simulink model "momentumBasedYoga"  (Simulink 8.8)
settings: Solver=FixedStepDiscrete  StartTime=0.0  StopTime="Config.SIMULATION_TIME "  FixedStep=Config.T_STEP  RelTol=1e-3  EnableMultiTasking=on
InitFcn:
  | cd(fileparts(which(bdroot)));
  | initMomentumBasedYoga;
StopFcn:
  | cd(fileparts(which(bdroot)));
  | stopMomentumBasedYoga;
undefined symbols (not defined in the file or in its folder): bVectorConstraints, Config, ConstraintsMatrix, Gain, Reg, ROBOT_DOF, ROBOT_DOF_FOR_SIMULINK, Sat, Sm
libraries: WBToolboxLibrary x89, simulink x4
(part 1 of 2)
settings Model: SuppressorTable=22 serialization::archive 11 0 6 0 0 0 11 0  Creator=daniele  LastModifiedBy=gnava
settings DataIOCC: SignalLoggingSaveFormat=Dataset
settings OptimizationCC: ExpressionDepthLimit=2147483647
settings DebuggingCC: SolverPrmCheckMsg=warning  AllowSymbolicDim=off
settings SFSimCC: SimParseCustomCode=off

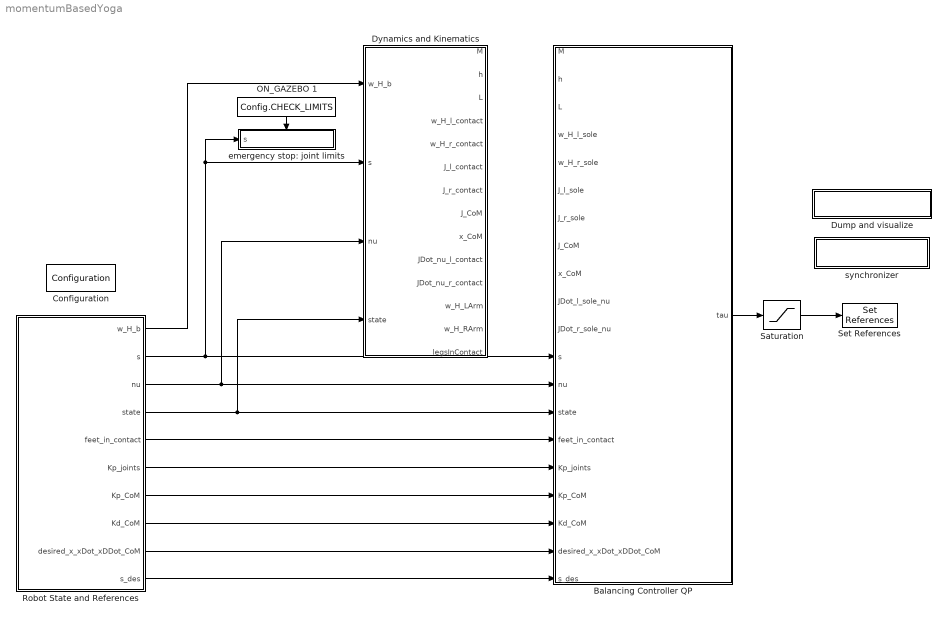
== system momentumBasedYoga ==
  Balancing Controller QP : Subsystem
  Configuration : WBToolboxLibrary/Utilities/Configuration  ConfigSource=Workspace  ConfigObject='WBTConfigRobot'  RobotName='icub'  UrdfFile='model.urdf'  ControlledJoints={'l_elbow','l_shoulder_pitch','torso_roll'}  ControlBoardsNames={'left_arm','right_arm','torso'}  LocalName='WBT'  GravityVector=[0,0,-9.81]
  Dump and visualize : Subsystem
      mask Display: disp('VISUALIZER')
  Dynamics and Kinematics : Subsystem
  ON_GAZEBO 1 : Constant  Value=Config.CHECK_LIMITS
  Robot State and References : Subsystem  Priority=-10
  Saturation : Saturate  UpperLimit=Sat.torque  LowerLimit=-Sat.torque
  Set References : WBToolboxLibrary/wholeBodyActuators/Set References  controlType=Torque  refSpeed=50
  emergency stop: joint limits : Subsystem
      mask Display: disp('EMERGENCY STOP')
  synchronizer : Subsystem
      mask Display: disp('SYNCHRONIZER')
  wires:
  Saturation/1 -> Set References/1
  ON_GAZEBO 1/1 -> emergency stop: joint limits/Enable
  Robot State and References/1(w_H_b) -> Dynamics and Kinematics/1(w_H_b)
  Robot State and References/2(s) -> Balancing Controller QP/12(s), emergency stop: joint limits/1(s), Dynamics and Kinematics/2(s)
  Robot State and References/3(nu) -> Balancing Controller QP/13(nu), Dynamics and Kinematics/3(nu)
  Robot State and References/4(state) -> Dynamics and Kinematics/4("state "), Balancing Controller QP/14(state)
  Robot State and References/5(feet_in_contact) -> Balancing Controller QP/15(feet_in_contact)
  Robot State and References/6(Kp_joints) -> Balancing Controller QP/16(Kp_joints)
  Robot State and References/7(Kp_CoM) -> Balancing Controller QP/17(Kp_CoM)
  Robot State and References/8(Kd_CoM) -> Balancing Controller QP/18(Kd_CoM)
  Robot State and References/9(desired_x_xDot_xDDot_CoM) -> Balancing Controller QP/19(desired_x_xDot_xDDot_CoM)
  Robot State and References/10(s_des) -> Balancing Controller QP/20(s_des)
  Balancing Controller QP/1("tau ") -> Saturation/1

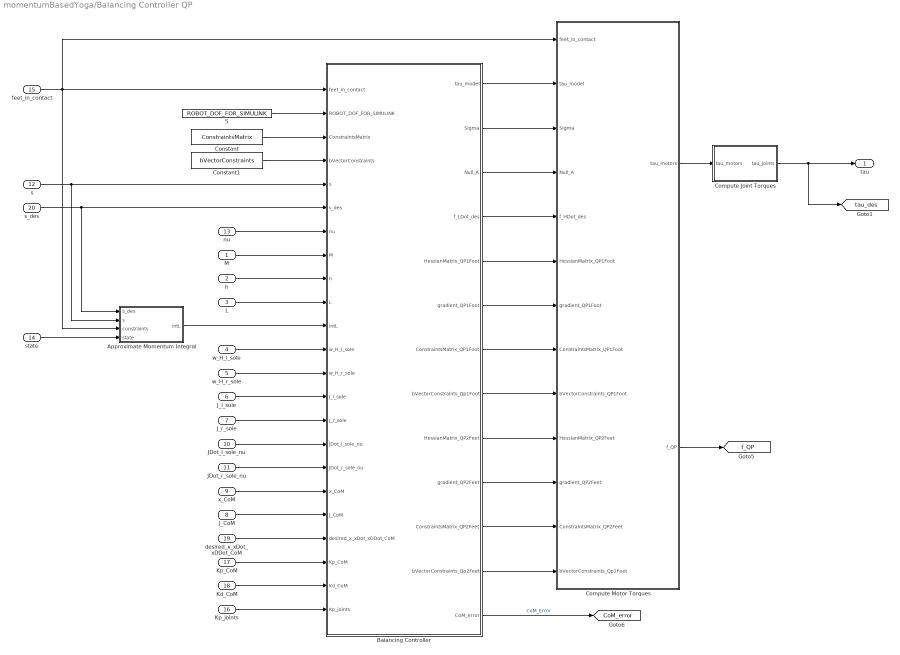
== system momentumBasedYoga/Balancing Controller QP ==
  M : Inport
  h : Inport  Port=2
  "L " : Inport  Port=3
  w_H_l_sole : Inport  Port=4
  w_H_r_sole : Inport  Port=5
  J_l_sole : Inport  Port=6
  J_r_sole : Inport  Port=7
  J_CoM : Inport  Port=8
  x_CoM : Inport  Port=9
  JDot_l_sole_nu : Inport  Port=10
  JDot_r_sole_nu : Inport  Port=11
  s : Inport  Port=12
  nu : Inport  Port=13
  state : Inport  Port=14
  feet_in_contact : Inport  Port=15
  Kp_joints : Inport  Port=16
  Kp_CoM : Inport  Port=17
  Kd_CoM : Inport  Port=18
  desired_x_xDot_xDDot_CoM : Inport  Port=19
  s_des : Inport  Port=20
  "    5" : Constant  Value=ROBOT_DOF_FOR_SIMULINK
  Approximate Momentum Integral : Subsystem
  "Balancing Controller " : MATLAB Function  TreatAsAtomicUnit=on
  Compute Joint Torques : Subsystem
  Compute Motor Torques : Subsystem
  Constant : Constant  Value=ConstraintsMatrix
  Constant1 : Constant  Value=bVectorConstraints
  "tau " : Outport
  tag scope: CoM_error=global, f_QP=global, tau_des=global
  wires:
  feet_in_contact/1 -> Compute Motor Torques/1(feet_in_contact), "Balancing Controller "/1(feet_in_contact), Approximate Momentum Integral/3(constraints)
  s/1 -> Approximate Momentum Integral/2(s), "Balancing Controller "/5(s)
  s_des/1 -> Approximate Momentum Integral/1(s_des), "Balancing Controller "/6(s_des)
  M/1 -> "Balancing Controller "/8(M)
  h/1 -> "Balancing Controller "/9(h)
  desired_x_xDot_xDDot_CoM/1 -> "Balancing Controller "/20(desired_x_xDot_xDDot_CoM)
  Kp_joints/1 -> "Balancing Controller "/23(Kp_joints)
  "L "/1 -> "Balancing Controller "/10(L)
  "    5"/1 -> "Balancing Controller "/2(ROBOT_DOF_FOR_SIMULINK)
  Constant/1 -> "Balancing Controller "/3(ConstraintsMatrix)
  Constant1/1 -> "Balancing Controller "/4(bVectorConstraints)
  nu/1 -> "Balancing Controller "/7(nu)
  Kp_CoM/1 -> "Balancing Controller "/21(Kp_CoM)
  Kd_CoM/1 -> "Balancing Controller "/22(Kd_CoM)
  w_H_r_sole/1 -> "Balancing Controller "/13(w_H_r_sole)
  w_H_l_sole/1 -> "Balancing Controller "/12(w_H_l_sole)
  J_l_sole/1 -> "Balancing Controller "/14(J_l_sole)
  J_r_sole/1 -> "Balancing Controller "/15(J_r_sole)
  Approximate Momentum Integral/1(intL) -> "Balancing Controller "/11(intL)
  JDot_l_sole_nu/1 -> "Balancing Controller "/16(JDot_l_sole_nu)
  JDot_r_sole_nu/1 -> "Balancing Controller "/17(JDot_r_sole_nu)
  J_CoM/1 -> "Balancing Controller "/19(J_CoM)
  x_CoM/1 -> "Balancing Controller "/18(x_CoM)
  state/1 -> Approximate Momentum Integral/4(state)
  Compute Motor Torques/1("tau_motors ") -> Compute Joint Torques/1(tau_motors)
  "Balancing Controller "/1(tau_model) -> Compute Motor Torques/2(tau_model)
  "Balancing Controller "/2(Sigma) -> Compute Motor Torques/3(Sigma)
  "Balancing Controller "/3(Null_A) -> Compute Motor Torques/4(Null_A)
  "Balancing Controller "/4(f_LDot_des) -> Compute Motor Torques/5(f_HDot_des)
  "Balancing Controller "/5(HessianMatrix_QP1Foot) -> Compute Motor Torques/6(HessianMatrix_QP1Foot)
  "Balancing Controller "/6(gradient_QP1Foot) -> Compute Motor Torques/7(gradient_QP1Foot)
  "Balancing Controller "/7(ConstraintsMatrix_QP1Foot) -> Compute Motor Torques/8(ConstraintsMatrix_QP1Foot)
  "Balancing Controller "/8(bVectorConstraints_Qp1Foot) -> Compute Motor Torques/9(bVectorConstraints_QP1Foot)
  "Balancing Controller "/9(HessianMatrix_QP2Feet) -> Compute Motor Torques/10(HessianMatrix_QP2Feet)
  "Balancing Controller "/10(gradient_QP2Feet) -> Compute Motor Torques/11(gradient_QP2Feet)
  "Balancing Controller "/11(ConstraintsMatrix_QP2Feet) -> Compute Motor Torques/12(ConstraintsMatrix_QP2Feet)
  "Balancing Controller "/12(bVectorConstraints_Qp2Feet) -> Compute Motor Torques/13(bVectorConstraints_Qp2Feet)
  "Balancing Controller "/13(CoM_error) -> [CoM_error]  "CoM_Error"
  Compute Motor Torques/2(f_QP) -> [f_QP]
  Compute Joint Torques/1(tau_joints) -> "tau "/1, [tau_des]

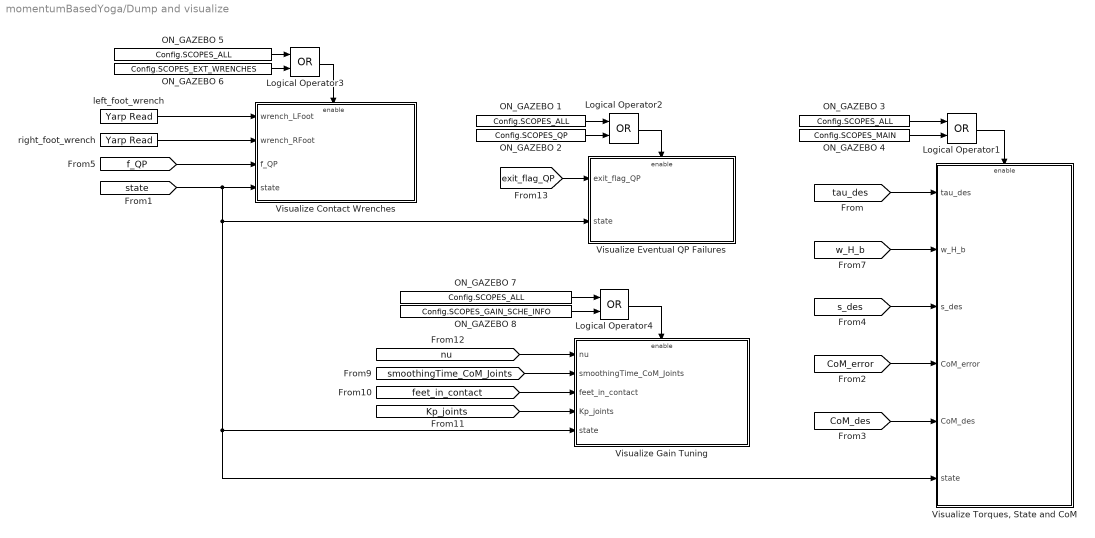
== system momentumBasedYoga/Dump and visualize ==
  Logical Operator{1..4} (4 alike) : Logic  Operator=OR  AllPortsSameDT=off  OutDataTypeStr=boolean
  ON_GAZEBO {1,3,5,7} (4 alike) : Constant  Value=Config.SCOPES_ALL
  ON_GAZEBO 2 : Constant  Value=Config.SCOPES_QP
  ON_GAZEBO 4 : Constant  Value=Config.SCOPES_MAIN
  ON_GAZEBO 6 : Constant  Value=Config.SCOPES_EXT_WRENCHES
  ON_GAZEBO 8 : Constant  Value=Config.SCOPES_GAIN_SCHE_INFO
  Visualize Contact Wrenches : Subsystem
  Visualize Eventual QP Failures : Subsystem
  "Visualize Gain Tuning  " : Subsystem
  "Visualize Torques, State and CoM" : Subsystem
  left_foot_wrench : WBToolboxLibrary/Utilities/Yarp Read  portName=Ports.WRENCH_LEFT_FOOT  signalSize=6  timeout=0.5  blocking=off  timestamp=off  autoconnect=on  errorOnConnection=on
  right_foot_wrench : WBToolboxLibrary/Utilities/Yarp Read  portName=Ports.WRENCH_RIGHT_FOOT  signalSize=6  timeout=0.5  blocking=off  timestamp=off  autoconnect=on  errorOnConnection=on
  wires:
  ON_GAZEBO 3/1 -> Logical Operator1/1
  ON_GAZEBO 4/1 -> Logical Operator1/2
  Logical Operator1/1 -> "Visualize Torques, State and CoM"/Enable
  [CoM_error] -> "Visualize Torques, State and CoM"/4(CoM_error)
  [s_des] -> "Visualize Torques, State and CoM"/3(s_des)
  [w_H_b] -> "Visualize Torques, State and CoM"/2(w_H_b)
  [tau_des] -> "Visualize Torques, State and CoM"/1(tau_des)
  [CoM_des] -> "Visualize Torques, State and CoM"/5(CoM_des)
  right_foot_wrench/1 -> Visualize Contact Wrenches/2(wrench_RFoot)
  [exit_flag_QP] -> Visualize Eventual QP Failures/1(exit_flag_QP)
  Logical Operator2/1 -> Visualize Eventual QP Failures/Enable
  ON_GAZEBO 1/1 -> Logical Operator2/1
  ON_GAZEBO 2/1 -> Logical Operator2/2
  ON_GAZEBO 5/1 -> Logical Operator3/1
  ON_GAZEBO 6/1 -> Logical Operator3/2
  [f_QP] -> Visualize Contact Wrenches/3(f_QP)
  ON_GAZEBO 7/1 -> Logical Operator4/1
  Logical Operator4/1 -> "Visualize Gain Tuning  "/Enable
  ON_GAZEBO 8/1 -> Logical Operator4/2
  [nu] -> "Visualize Gain Tuning  "/1(nu)
  [Kp_joints] -> "Visualize Gain Tuning  "/4(Kp_joints)
  [feet_in_contact] -> "Visualize Gain Tuning  "/3(feet_in_contact)
  [smoothingTime_CoM_Joints] -> "Visualize Gain Tuning  "/2(smoothingTime_CoM_Joints)
  [state] -> "Visualize Torques, State and CoM"/6(state), "Visualize Gain Tuning  "/5(state), Visualize Eventual QP Failures/2(state), Visualize Contact Wrenches/4(state)
  Logical Operator3/1 -> Visualize Contact Wrenches/Enable
  left_foot_wrench/1 -> Visualize Contact Wrenches/1(wrench_LFoot)

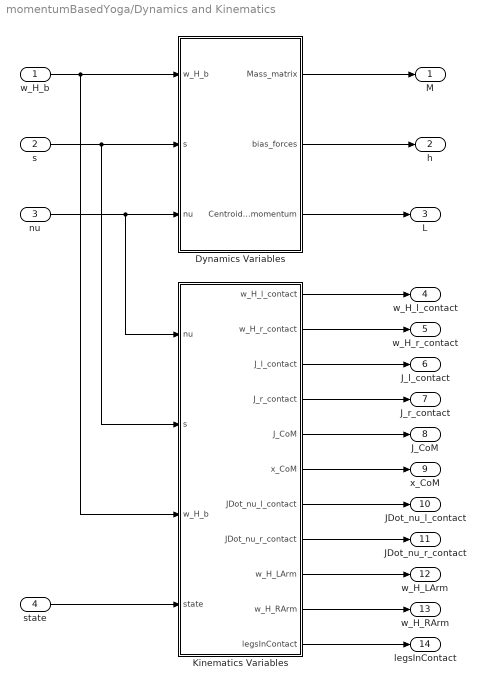
== system momentumBasedYoga/Dynamics and Kinematics ==
  w_H_b : Inport
  s : Inport  Port=2
  nu : Inport  Port=3
  "state " : Inport  Port=4
  Dynamics Variables : Subsystem
  Kinematics Variables : Subsystem
  M : Outport
  h : Outport  Port=2
  L : Outport  Port=3
  w_H_l_contact : Outport  Port=4
  w_H_r_contact : Outport  Port=5
  J_l_contact : Outport  Port=6
  J_r_contact : Outport  Port=7
  J_CoM : Outport  Port=8
  x_CoM : Outport  Port=9
  JDot_nu_l_contact : Outport  Port=10
  JDot_nu_r_contact : Outport  Port=11
  w_H_LArm : Outport  Port=12
  w_H_RArm : Outport  Port=13
  legsInContact : Outport  Port=14
  wires:
  Dynamics Variables/1(Mass_matrix) -> M/1
  Dynamics Variables/2(bias_forces) -> h/1
  Dynamics Variables/3(Centroidal_momentum) -> L/1
  Kinematics Variables/4(J_r_contact) -> J_r_contact/1
  Kinematics Variables/3(J_l_contact) -> J_l_contact/1
  "state "/1 -> Kinematics Variables/4("state ")
  Kinematics Variables/7(JDot_nu_l_contact) -> JDot_nu_l_contact/1
  Kinematics Variables/8(JDot_nu_r_contact) -> JDot_nu_r_contact/1
  Kinematics Variables/10(w_H_RArm) -> w_H_RArm/1
  Kinematics Variables/5(J_CoM) -> J_CoM/1
  Kinematics Variables/1(w_H_l_contact) -> w_H_l_contact/1
  w_H_b/1 -> Kinematics Variables/3(w_H_b), Dynamics Variables/1(w_H_b)
  Kinematics Variables/6(x_CoM) -> x_CoM/1
  Kinematics Variables/2(w_H_r_contact) -> w_H_r_contact/1
  nu/1 -> Kinematics Variables/1(nu), Dynamics Variables/3(nu)
  Kinematics Variables/11(legsInContact) -> legsInContact/1
  Kinematics Variables/9(w_H_LArm) -> w_H_LArm/1
  s/1 -> Kinematics Variables/2(s), Dynamics Variables/2(s)

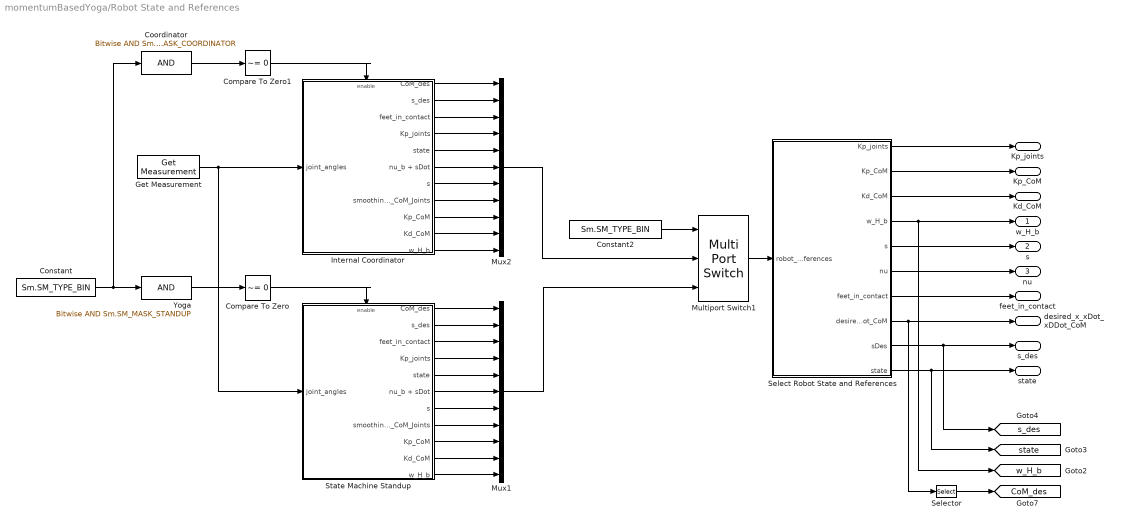
== system momentumBasedYoga/Robot State and References ==
  Compare To Zero : simulink/Logic and Bit Operations/Compare To Zero  relop=~=  OutDataTypeStr=boolean
  Compare To Zero1 : simulink/Logic and Bit Operations/Compare To Zero  relop=~=  OutDataTypeStr=boolean
  Constant : Constant  Priority=-10  Value=Sm.SM_TYPE_BIN  OutDataTypeStr=uint8
  Constant2 : Constant  Priority=-10  Value=Sm.SM_TYPE_BIN  OutDataTypeStr=uint8
  Coordinator : simulink/Logic and Bit Operations/Bitwise Operator  logicop=AND  UseBitMask=on  BitMask=Sm.SM_MASK_COORDINATOR  BitMaskRealWorld=Stored Integer
  Get Measurement : WBToolboxLibrary/wholeBodyStates/Get Measurement  measuredType=Joints Position
  Internal Coordinator : Subsystem
  Multiport Switch1 : MultiPortSwitch  DataPortOrder=Specify indices  DataPortIndices={1, 2}
  Mux1 : Mux  Inputs=11
  Mux2 : Mux  Inputs=11
  Select Robot State and References : Subsystem
  Selector : Selector  NumberOfDimensions=2  InputPortWidth=3  IndexOptions=Index vector (dialog),Index vector (dialog)  Indices=[1 2 3],[1]  OutputSizes=1,1
  State Machine Standup : Subsystem  Priority=-100
  Yoga : simulink/Logic and Bit Operations/Bitwise Operator  logicop=AND  UseBitMask=on  BitMask=Sm.SM_MASK_STANDUP  BitMaskRealWorld=Stored Integer
  w_H_b : Outport
  s : Outport  Port=2
  nu : Outport  Port=3
  state : Outport  Port=4
  feet_in_contact : Outport  Port=5
  Kp_joints : Outport  Port=6
  Kp_CoM : Outport  Port=7
  Kd_CoM : Outport  Port=8
  desired_x_xDot_xDDot_CoM : Outport  Port=9
  s_des : Outport  Port=10
  tag scope: CoM_des=global, s_des=global, state=global, w_H_b=global
  wires:
  Constant/1 -> Yoga/1, Coordinator/1
  State Machine Standup/3(feet_in_contact) -> Mux1/3
  State Machine Standup/2(s_des) -> Mux1/2
  State Machine Standup/1(CoM_des) -> Mux1/1
  Internal Coordinator/1(CoM_des) -> Mux2/1
  Internal Coordinator/2(s_des) -> Mux2/2
  Internal Coordinator/3(feet_in_contact) -> Mux2/3
  State Machine Standup/4(Kp_joints) -> Mux1/4
  Internal Coordinator/4(Kp_joints) -> Mux2/4
  State Machine Standup/5(state) -> Mux1/5
  Internal Coordinator/5(state) -> Mux2/5
  Internal Coordinator/6(nu_b + sDot) -> Mux2/6
  Internal Coordinator/7(s) -> Mux2/7
  State Machine Standup/6(nu_b + sDot) -> Mux1/6
  State Machine Standup/7(s) -> Mux1/7
  Coordinator/1 -> Compare To Zero1/1
  Yoga/1 -> Compare To Zero/1
  Compare To Zero/1 -> State Machine Standup/Enable
  Compare To Zero1/1 -> Internal Coordinator/Enable
  Internal Coordinator/8(smoothingTime_CoM_Joints) -> Mux2/8
  State Machine Standup/8(smoothingTime_CoM_Joints) -> Mux1/8
  State Machine Standup/9(Kp_CoM) -> Mux1/9
  State Machine Standup/10(Kd_CoM) -> Mux1/10
  Internal Coordinator/9(Kp_CoM) -> Mux2/9
  Internal Coordinator/10(Kd_CoM) -> Mux2/10
  Constant2/1 -> Multiport Switch1/1
  Get Measurement/1 -> Internal Coordinator/1(joint_angles), State Machine Standup/1(joint_angles)
  State Machine Standup/11(w_H_b) -> Mux1/11
  Internal Coordinator/11(w_H_b) -> Mux2/11
  Mux2/1 -> Multiport Switch1/2
  Mux1/1 -> Multiport Switch1/3
  Multiport Switch1/1 -> Select Robot State and References/1(robot_state_and_references)
  Select Robot State and References/1(Kp_joints) -> Kp_joints/1
  Select Robot State and References/2(Kp_CoM) -> Kp_CoM/1
  Select Robot State and References/3(Kd_CoM) -> Kd_CoM/1
  Select Robot State and References/4(w_H_b) -> w_H_b/1, [w_H_b]
  Select Robot State and References/5(s) -> s/1
  Select Robot State and References/6(nu) -> nu/1
  Select Robot State and References/7(feet_in_contact) -> feet_in_contact/1
  Select Robot State and References/8(desired_x_xDot_xDDot_CoM) -> desired_x_xDot_xDDot_CoM/1, Selector/1
  Select Robot State and References/9(sDes) -> s_des/1, [s_des]
  Select Robot State and References/10(state) -> state/1, [state]
  Selector/1 -> [CoM_des]

== system momentumBasedYoga/emergency stop: joint limits ==
  s : Inport
  Enable : EnablePort
  Assertion : Assertion
  Get Limits : WBToolboxLibrary/wholeBodyStates/Get Limits  limitsSource=ControlBoard  limitsType=Position
  MATLAB Function : MATLAB Function  TreatAsAtomicUnit=on
  index1 : Constant  Value=0.01  VectorParams1D=off
  wires:
  Get Limits/1 -> MATLAB Function/1(umin)
  Get Limits/2 -> MATLAB Function/2(umax)
  index1/1 -> MATLAB Function/4(tol)
  s/1 -> MATLAB Function/3(u)
  MATLAB Function/1(inRange) -> Assertion/1

== system momentumBasedYoga/synchronizer ==
  GAZEBO_SYNCHRONIZER : Subsystem
  Logical Operator : Logic  Operator=NOT  AllPortsSameDT=off  OutDataTypeStr=boolean
  "ON_GAZEBO " : Constant  Value=Config.ON_GAZEBO
  REAL_TIME_SYNC : Subsystem
  wires:
  Logical Operator/1 -> REAL_TIME_SYNC/Enable
  "ON_GAZEBO "/1 -> GAZEBO_SYNCHRONIZER/Enable, Logical Operator/1

== system momentumBasedYoga/Balancing Controller QP/Approximate Momentum Integral ==
  s_des : Inport
  s : Inport  Port=2
  constraints : Inport  Port=3
  state : Inport  Port=4
  Centroidal Momentum : WBToolboxLibrary/wholeBodyModel/Dynamics/Centroidal Momentum
  Compute base to fixed link transform : Subsystem
  Jacobian : WBToolboxLibrary/wholeBodyModel/Jacobians/Jacobian  frameName=Frames.LEFT_FOOT
  Jacobian1 : WBToolboxLibrary/wholeBodyModel/Jacobians/Jacobian  frameName=Frames.RIGHT_FOOT
  References for L : MATLAB Function  TreatAsAtomicUnit=on
  Sum : Sum  Inputs=|-+
  Switch : Switch  Criteria=u2 > Threshold  Threshold=0.1
  choose base to world transform : MATLAB Function  TreatAsAtomicUnit=on
  inertial : WBToolboxLibrary/Utilities/Yarp Read  portName=Ports.IMU  signalSize=12  timeout=0.5  blocking=off  timestamp=off  autoconnect=on  errorOnConnection=on
  intL : Outport
  wires:
  s_des/1 -> Compute base to fixed link transform/1(s), Centroidal Momentum/2, Jacobian/2, Sum/1, Jacobian1/2
  s/1 -> Sum/2
  Sum/1 -> Centroidal Momentum/4, References for L/1(s_err)
  References for L/1(nu_b_equivalent) -> Centroidal Momentum/3
  Jacobian/1 -> References for L/2(JL)
  Centroidal Momentum/1 -> intL/1
  Jacobian1/1 -> References for L/3(JR)
  constraints/1 -> References for L/4(activeFeetConstraints)
  state/1 -> choose base to world transform/1(state)
  choose base to world transform/1(booleanState) -> Switch/2
  Switch/1 -> Centroidal Momentum/1, Jacobian/1, Jacobian1/1
  inertial/1 -> Compute base to fixed link transform/2(inertial)
  Compute base to fixed link transform/1(fixed_LFoot_H_b) -> Switch/1
  Compute base to fixed link transform/2(fixed_RFoot_H_b) -> Switch/3

== system momentumBasedYoga/Balancing Controller QP/Compute Joint Torques ==
  tau_motors : Inport
  " " : Constant  Value=Config.USE_MOTOR_REFLECTED_INERTIA
  "(transpose(T*Gamma))^{-1}*I_m*(T*Gamma)^{-1}" : MATLAB Function  TreatAsAtomicUnit=on
  Add : Sum  Inputs=-+
  Feedforward : Gain  Gain=Config.K_ff
  Get Measurement : WBToolboxLibrary/wholeBodyStates/Get Measurement  measuredType=Joints Acceleration
  Product : Product  Multiplication=Matrix(*)
  Switch : Switch  Criteria=u2 > Threshold
  tau_joints : Outport
  wires:
  Get Measurement/1 -> Product/2
  Product/1 -> Feedforward/1
  Feedforward/1 -> Add/1
  Add/1 -> Switch/1
  " "/1 -> Switch/2
  Switch/1 -> tau_joints/1
  tau_motors/1 -> Add/2, Switch/3
  "(transpose(T*Gamma))^{-1}*I_m*(T*Gamma)^{-1}"/1(reflectedInertia) -> Product/1

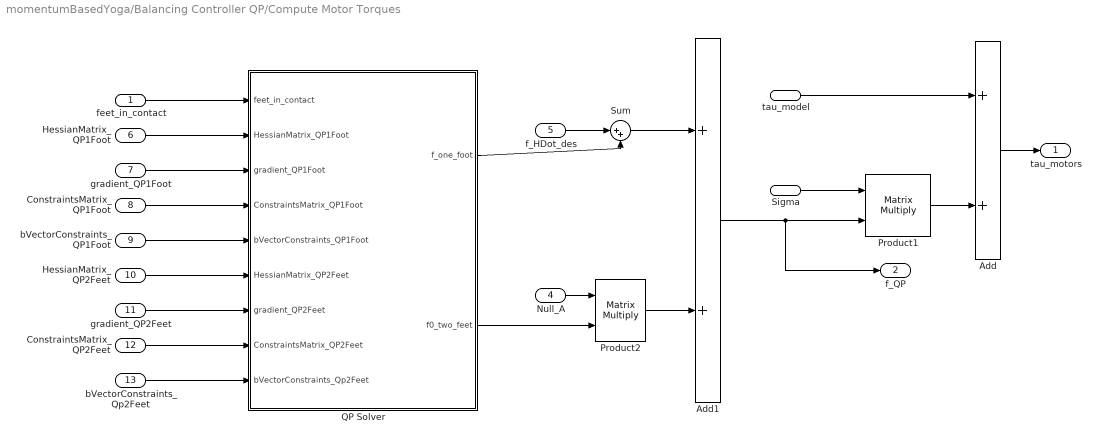
== system momentumBasedYoga/Balancing Controller QP/Compute Motor Torques ==
  feet_in_contact : Inport
  tau_model : Inport  Port=2
  Sigma : Inport  Port=3
  Null_A : Inport  Port=4
  f_HDot_des : Inport  Port=5
  HessianMatrix_QP1Foot : Inport  Port=6
  gradient_QP1Foot : Inport  Port=7
  ConstraintsMatrix_QP1Foot : Inport  Port=8
  bVectorConstraints_QP1Foot : Inport  Port=9
  HessianMatrix_QP2Feet : Inport  Port=10
  gradient_QP2Feet : Inport  Port=11
  ConstraintsMatrix_QP2Feet : Inport  Port=12
  bVectorConstraints_Qp2Feet : Inport  Port=13
  Add : Sum
  Add1 : Sum
  Product1 : Product  Multiplication=Matrix(*)
  Product2 : Product  Multiplication=Matrix(*)
  QP Solver : Subsystem
  Sum : Sum  Inputs=|++
  "tau_motors " : Outport
  f_QP : Outport  Port=2
  wires:
  Null_A/1 -> Product2/1
  QP Solver/1(f_one_foot) -> Sum/2
  Product1/1 -> Add/2
  tau_model/1 -> Add/1
  Add/1 -> "tau_motors "/1
  Add1/1 -> f_QP/1, Product1/2
  Sum/1 -> Add1/1
  Product2/1 -> Add1/2
  Sigma/1 -> Product1/1
  QP Solver/2(f0_two_feet) -> Product2/2
  gradient_QP1Foot/1 -> QP Solver/3(gradient_QP1Foot)
  ConstraintsMatrix_QP2Feet/1 -> QP Solver/8(ConstraintsMatrix_QP2Feet)
  feet_in_contact/1 -> QP Solver/1(feet_in_contact)
  bVectorConstraints_QP1Foot/1 -> QP Solver/5(bVectorConstraints_QP1Foot)
  HessianMatrix_QP1Foot/1 -> QP Solver/2(HessianMatrix_QP1Foot)
  ConstraintsMatrix_QP1Foot/1 -> QP Solver/4(ConstraintsMatrix_QP1Foot)
  gradient_QP2Feet/1 -> QP Solver/7(gradient_QP2Feet)
  HessianMatrix_QP2Feet/1 -> QP Solver/6(HessianMatrix_QP2Feet)
  bVectorConstraints_Qp2Feet/1 -> QP Solver/9(bVectorConstraints_Qp2Feet)
  f_HDot_des/1 -> Sum/1

== system momentumBasedYoga/Dump and visualize/Visualize Contact Wrenches ==
  wrench_LFoot : Inport
  wrench_RFoot : Inport  Port=2
  f_QP : Inport  Port=3
  state : Inport  Port=4
  Enable : EnablePort
  Demux{1..5} (5 alike) : Demux  Outputs=2
  Left Foot Forces : Scope  NumInputPorts=4
  Left Foot Moments : Scope  NumInputPorts=4
  Right Foot Forces : Scope  NumInputPorts=4
  Right Foot Moments : Scope  NumInputPorts=4
  Sum{1..4} (4 alike) : Sum  Inputs=+-|
  wires:
  f_QP/1 -> Demux1/1
  Demux1/1 -> Demux2/1  "LFoot_wrench"
  wrench_LFoot/1 -> Demux3/1  "LFoot_wrench"
  Sum2/1 -> Left Foot Moments/3  "moments error"
  Sum1/1 -> Left Foot Forces/3  "forces error"
  Demux2/1 -> Sum1/1, Left Foot Forces/1  "desired forces"
  Demux2/2 -> Sum2/1, Left Foot Moments/1  "desired moments"
  Demux3/1 -> Sum1/2, Left Foot Forces/2  "measured forces"
  Demux3/2 -> Left Foot Moments/2, Sum2/2  "measured moments"
  Demux4/2 -> Sum4/1, Right Foot Moments/1  "desired moments"
  Demux5/1 -> Sum3/2, Right Foot Forces/2  "measured forces"
  Demux4/1 -> Sum3/1, Right Foot Forces/1  "desired forces"
  Demux5/2 -> Right Foot Moments/2, Sum4/2  "measured moments"
  Sum3/1 -> Right Foot Forces/3  "forces error"
  Sum4/1 -> Right Foot Moments/3  "moments error"
  Demux1/2 -> Demux4/1  "RFoot_wrench"
  state/1 -> Left Foot Forces/4, Left Foot Moments/4, Right Foot Forces/4, Right Foot Moments/4
  wrench_RFoot/1 -> Demux5/1  "RFoot_wrench"

== system momentumBasedYoga/Dump and visualize/Visualize Eventual QP Failures ==
  exit_flag_QP : Inport
  state : Inport  Port=2
  Enable : EnablePort
  "QP status (0: no failure, 1: not using)" : Scope  NumInputPorts=2
  wires:
  exit_flag_QP/1 -> "QP status (0: no failure, 1: not using)"/1
  state/1 -> "QP status (0: no failure, 1: not using)"/2

== system momentumBasedYoga/Dump and visualize/Visualize Gain Tuning   ==
  nu : Inport
  smoothingTime_CoM_Joints : Inport  Port=2
  feet_in_contact : Inport  Port=3
  Kp_joints : Inport  Port=4
  state : Inport  Port=5
  Enable : EnablePort
  Demux : Demux  Outputs=2
  DoFs converter : WBToolboxLibrary/Utilities/DoFs converter  yarp2WBIOption=From YARP to WBI
  DoFs converter1 : WBToolboxLibrary/Utilities/DoFs converter  yarp2WBIOption=From YARP to WBI
  Feet in Contact : Scope
  Gain : Gain  Gain=180/pi
  Gain1 : Gain  Gain=180/pi
  Kp Joints : Scope  NumInputPorts=6
  Selector1 : Selector  InputPortWidth=6+ROBOT_DOF  IndexOptions=Index vector (dialog)  Indices=[7:6+ROBOT_DOF]  OutputSizes=1
  Selector2 : Selector  InputPortWidth=6+ROBOT_DOF  IndexOptions=Index vector (dialog)  Indices=[1:6]  OutputSizes=1
  nu_base : Scope  NumInputPorts=3
  sDot : Scope  NumInputPorts=6
  smoothingTime CoM and Joints : Scope  NumInputPorts=2
  wires:
  state/1 -> sDot/6, nu_base/3, Kp Joints/6, smoothingTime CoM and Joints/2
  feet_in_contact/1 -> Feet in Contact/1
  Kp_joints/1 -> DoFs converter/1
  smoothingTime_CoM_Joints/1 -> smoothingTime CoM and Joints/1
  DoFs converter/4 -> Kp Joints/4  "left_leg"
  DoFs converter/5 -> Kp Joints/5  "right_leg"
  DoFs converter/3 -> Kp Joints/3  "right_arm"
  DoFs converter/1 -> Kp Joints/1  "torso"
  DoFs converter/2 -> Kp Joints/2  "left_arm"
  Selector1/1 -> Gain/1
  DoFs converter1/4 -> sDot/4  "left_leg"
  DoFs converter1/3 -> sDot/3  "right_arm"
  DoFs converter1/1 -> sDot/1  "torso"
  DoFs converter1/2 -> sDot/2  "left_arm"
  nu/1 -> Selector2/1, Selector1/1
  Selector2/1 -> Demux/1
  Demux/1 -> nu_base/1  "v_b"
  Demux/2 -> Gain1/1
  Gain/1 -> DoFs converter1/1
  Gain1/1 -> nu_base/2  "omega_b"
  DoFs converter1/5 -> sDot/5  "right_leg"

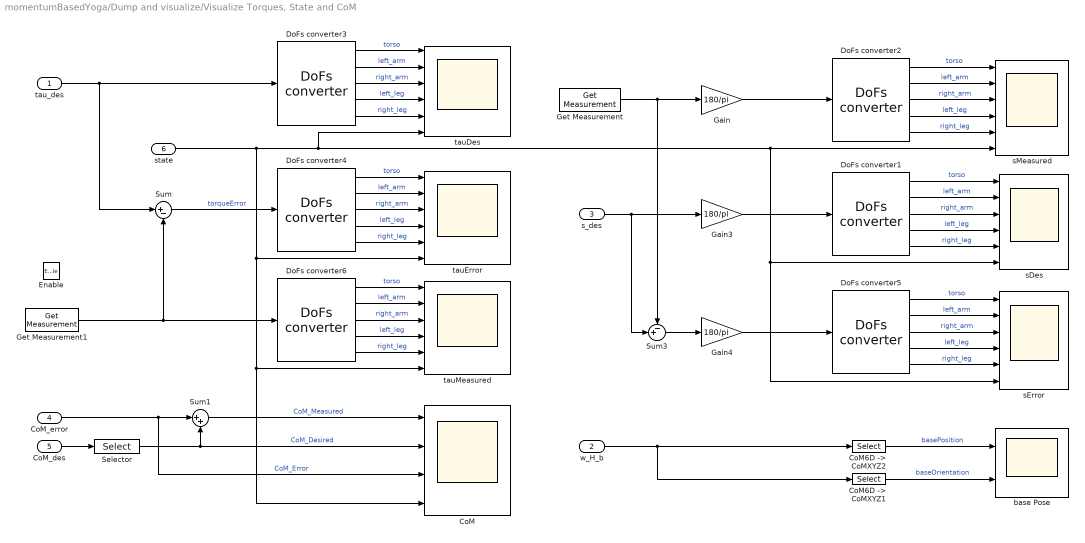
== system momentumBasedYoga/Dump and visualize/Visualize Torques, State and CoM ==
  tau_des : Inport
  w_H_b : Inport  Port=2
  s_des : Inport  Port=3
  CoM_error : Inport  Port=4
  CoM_des : Inport  Port=5
  state : Inport  Port=6
  Enable : EnablePort
  CoM : Scope  NumInputPorts=4
  "CoM6D ->  CoMXYZ1" : Selector  NumberOfDimensions=2  InputPortWidth=7  IndexOptions=Index vector (dialog),Index vector (dialog)  Indices=[1 2 3],[1 2 3]  OutputSizes=1,1
  "CoM6D ->  CoMXYZ2" : Selector  NumberOfDimensions=2  InputPortWidth=7  IndexOptions=Index vector (dialog),Index vector (dialog)  Indices=[1 2 3],[4]  OutputSizes=1,1
  DoFs converter{1..6} (6 alike) : WBToolboxLibrary/Utilities/DoFs converter  yarp2WBIOption=From YARP to WBI
  Gain : Gain  Gain=180/pi
  Gain3 : Gain  Gain=180/pi
  Gain4 : Gain  Gain=180/pi
  Get Measurement : WBToolboxLibrary/wholeBodyStates/Get Measurement  measuredType=Joints Position
  Get Measurement1 : WBToolboxLibrary/wholeBodyStates/Get Measurement  measuredType=Joints Torque
  Selector : Selector  NumberOfDimensions=2  IndexOptions=Index vector (dialog),Index vector (dialog)  Indices=[1:3],1  OutputSizes=1,1
  Sum : Sum  Inputs=|+-
  Sum1 : Sum  Inputs=|++
  Sum3 : Sum  Inputs=-+|
  base Pose : Scope  NumInputPorts=2
  sDes : Scope  NumInputPorts=6
  sError : Scope  NumInputPorts=6
  sMeasured : Scope  NumInputPorts=6
  tauDes : Scope  NumInputPorts=6
  tauError : Scope  NumInputPorts=6
  tauMeasured : Scope  NumInputPorts=6
  wires:
  CoM_error/1 -> Sum1/1, CoM/3  "CoM_Error"
  CoM_des/1 -> Selector/1
  Gain/1 -> DoFs converter2/1
  Sum1/1 -> CoM/1  "CoM_Measured"
  Get Measurement/1 -> Gain/1, Sum3/1
  DoFs converter2/5 -> sMeasured/5  "right_leg"
  DoFs converter2/1 -> sMeasured/1  "torso"
  DoFs converter2/2 -> sMeasured/2  "left_arm"
  DoFs converter2/4 -> sMeasured/4  "left_leg"
  DoFs converter2/3 -> sMeasured/3  "right_arm"
  tau_des/1 -> DoFs converter3/1, Sum/1
  Get Measurement1/1 -> DoFs converter6/1, Sum/2
  DoFs converter3/5 -> tauDes/5  "right_leg"
  DoFs converter3/1 -> tauDes/1  "torso"
  DoFs converter3/2 -> tauDes/2  "left_arm"
  DoFs converter3/4 -> tauDes/4  "left_leg"
  DoFs converter3/3 -> tauDes/3  "right_arm"
  DoFs converter4/5 -> tauError/5  "right_leg"
  DoFs converter4/1 -> tauError/1  "torso"
  DoFs converter4/2 -> tauError/2  "left_arm"
  DoFs converter4/4 -> tauError/4  "left_leg"
  DoFs converter4/3 -> tauError/3  "right_arm"
  Sum/1 -> DoFs converter4/1  "torqueError"
  DoFs converter6/5 -> tauMeasured/5  "right_leg"
  DoFs converter6/1 -> tauMeasured/1  "torso"
  DoFs converter6/2 -> tauMeasured/2  "left_arm"
  DoFs converter6/4 -> tauMeasured/4  "left_leg"
  DoFs converter6/3 -> tauMeasured/3  "right_arm"
  s_des/1 -> Sum3/2, Gain3/1
  Gain3/1 -> DoFs converter1/1
  DoFs converter1/5 -> sDes/5  "right_leg"
  DoFs converter1/1 -> sDes/1  "torso"
  DoFs converter1/2 -> sDes/2  "left_arm"
  DoFs converter1/4 -> sDes/4  "left_leg"
  DoFs converter1/3 -> sDes/3  "right_arm"
  Gain4/1 -> DoFs converter5/1
  DoFs converter5/5 -> sError/5  "right_leg"
  DoFs converter5/1 -> sError/1  "torso"
  DoFs converter5/2 -> sError/2  "left_arm"
  DoFs converter5/4 -> sError/4  "left_leg"
  DoFs converter5/3 -> sError/3  "right_arm"
  Sum3/1 -> Gain4/1
  Selector/1 -> Sum1/2, CoM/2  "CoM_Desired"
  state/1 -> sError/6, sDes/6, sMeasured/6, tauDes/6, CoM/4, tauMeasured/6, tauError/6
  w_H_b/1 -> "CoM6D ->  CoMXYZ2"/1, "CoM6D ->  CoMXYZ1"/1
  "CoM6D ->  CoMXYZ2"/1 -> base Pose/1  "basePosition"
  "CoM6D ->  CoMXYZ1"/1 -> base Pose/2  "baseOrientation"

== system momentumBasedYoga/Dynamics and Kinematics/Dynamics Variables ==
  w_H_b : Inport
  s : Inport  Port=2
  nu : Inport  Port=3
  Add Motors Reflected Inertia : Subsystem
  Centroidal Momentum : WBToolboxLibrary/wholeBodyModel/Dynamics/Centroidal Momentum
  "CoM6D ->  CoMXYZ1" : Selector  InputPortWidth=6+ROBOT_DOF  IndexOptions=Index vector (dialog)  Indices=[7:6+ROBOT_DOF]  OutputSizes=1
  "CoM6D ->  CoMXYZ2" : Selector  InputPortWidth=6+ROBOT_DOF  IndexOptions=Index vector (dialog)  Indices=[1 2 3 4 5 6]  OutputSizes=1
  Get Bias Forces : WBToolboxLibrary/wholeBodyModel/Dynamics/Get Bias Forces
  Mass Matrix : WBToolboxLibrary/wholeBodyModel/Dynamics/Mass Matrix
  Mass_matrix : Outport
  bias_forces : Outport  Port=2
  Centroidal_momentum : Outport  Port=3
  wires:
  Centroidal Momentum/1 -> Centroidal_momentum/1
  Get Bias Forces/1 -> bias_forces/1
  w_H_b/1 -> Centroidal Momentum/1, Get Bias Forces/1, Mass Matrix/1
  s/1 -> Centroidal Momentum/2, Get Bias Forces/2, Mass Matrix/2
  "CoM6D ->  CoMXYZ2"/1 -> Centroidal Momentum/3, Get Bias Forces/3
  "CoM6D ->  CoMXYZ1"/1 -> Centroidal Momentum/4, Get Bias Forces/4
  nu/1 -> "CoM6D ->  CoMXYZ1"/1, "CoM6D ->  CoMXYZ2"/1
  Mass Matrix/1 -> Add Motors Reflected Inertia/1(M)
  Add Motors Reflected Inertia/1(M_with_motor_inertia) -> Mass_matrix/1

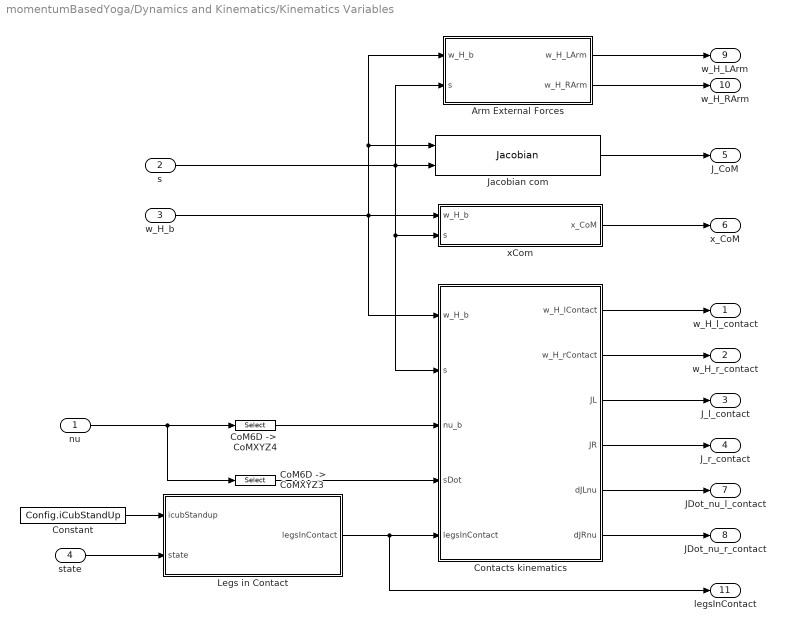
== system momentumBasedYoga/Dynamics and Kinematics/Kinematics Variables ==
  nu : Inport
  s : Inport  Port=2
  w_H_b : Inport  Port=3
  "state " : Inport  Port=4
  Arm External Forces : Subsystem
  "CoM6D ->  CoMXYZ3" : Selector  InputPortWidth=6+ROBOT_DOF  IndexOptions=Index vector (dialog)  Indices=[7:6+ROBOT_DOF]  OutputSizes=1
  "CoM6D ->  CoMXYZ4" : Selector  InputPortWidth=6+ROBOT_DOF  IndexOptions=Index vector (dialog)  Indices=[1 2 3 4 5 6]  OutputSizes=1
  Constant : Constant  Value=Config.iCubStandUp
  Contacts kinematics : Subsystem
  Jacobian com : WBToolboxLibrary/wholeBodyModel/Jacobians/Jacobian  frameName=Frames.COM
  Legs in Contact : MATLAB Function  TreatAsAtomicUnit=on
  xCom : Subsystem
  w_H_l_contact : Outport
  w_H_r_contact : Outport  Port=2
  J_l_contact : Outport  Port=3
  J_r_contact : Outport  Port=4
  J_CoM : Outport  Port=5
  x_CoM : Outport  Port=6
  JDot_nu_l_contact : Outport  Port=7
  JDot_nu_r_contact : Outport  Port=8
  w_H_LArm : Outport  Port=9
  w_H_RArm : Outport  Port=10
  legsInContact : Outport  Port=11
  wires:
  nu/1 -> "CoM6D ->  CoMXYZ3"/1, "CoM6D ->  CoMXYZ4"/1
  w_H_b/1 -> Contacts kinematics/1(w_H_b), xCom/1(w_H_b), Arm External Forces/1(w_H_b), Jacobian com/1
  s/1 -> Arm External Forces/2(s), Jacobian com/2, Contacts kinematics/2(s), xCom/2(s)
  Jacobian com/1 -> J_CoM/1
  xCom/1(x_CoM) -> x_CoM/1
  "state "/1 -> Legs in Contact/2(state)
  Constant/1 -> Legs in Contact/1(icubStandup)
  "CoM6D ->  CoMXYZ3"/1 -> Contacts kinematics/4(sDot)
  "CoM6D ->  CoMXYZ4"/1 -> Contacts kinematics/3(nu_b)
  Legs in Contact/1(legsInContact) -> legsInContact/1, Contacts kinematics/5(legsInContact)
  Contacts kinematics/1(w_H_lContact) -> w_H_l_contact/1
  Contacts kinematics/2(w_H_rContact) -> w_H_r_contact/1
  Contacts kinematics/5(dJLnu) -> JDot_nu_l_contact/1
  Contacts kinematics/6(dJRnu) -> JDot_nu_r_contact/1
  Contacts kinematics/3(JL) -> J_l_contact/1
  Contacts kinematics/4(JR) -> J_r_contact/1
  Arm External Forces/1(w_H_LArm) -> w_H_LArm/1
  Arm External Forces/2(w_H_RArm) -> w_H_RArm/1

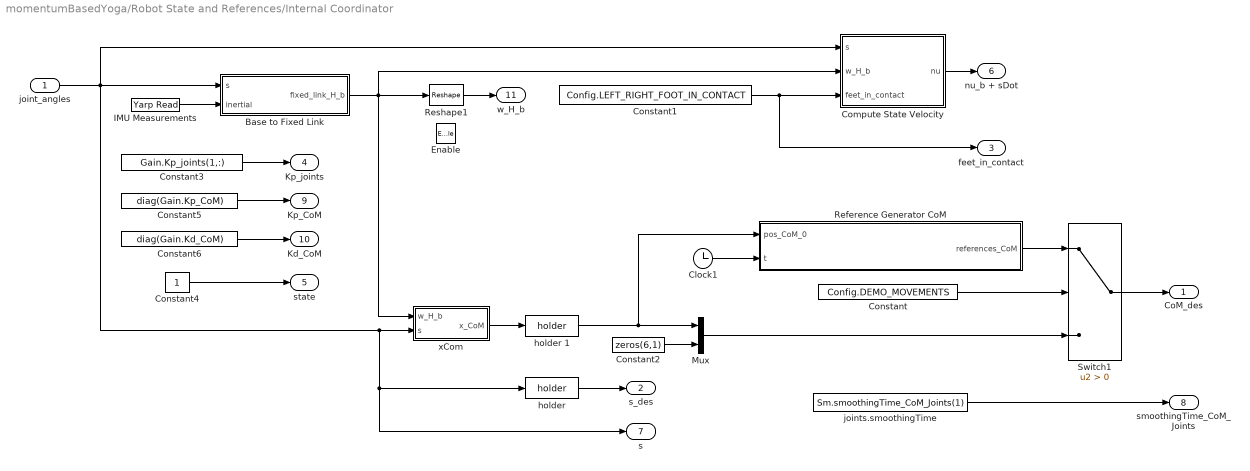
== system momentumBasedYoga/Robot State and References/Internal Coordinator ==
  joint_angles : Inport
  Enable : EnablePort
  Base to Fixed Link : Subsystem
  Clock1 : Clock
  Compute State Velocity : Subsystem
  Constant : Constant  Value=Config.DEMO_MOVEMENTS
  Constant1 : Constant  Value=Config.LEFT_RIGHT_FOOT_IN_CONTACT
  Constant2 : Constant  Value=zeros(6,1)
  Constant3 : Constant  Value=Gain.Kp_joints(1,:)
  Constant4 : Constant
  Constant5 : Constant  Value=diag(Gain.Kp_CoM)
  Constant6 : Constant  Value=diag(Gain.Kd_CoM)
  IMU Measurements : WBToolboxLibrary/Utilities/Yarp Read  portName=Ports.IMU  signalSize=12  timeout=0.5  blocking=off  timestamp=off  autoconnect=on  errorOnConnection=on
  Mux : Mux  Inputs=2
  Reference Generator CoM : MATLAB Function  TreatAsAtomicUnit=on
  Reshape1 : Reshape  OutputDimensions=[4;4]
  Switch1 : Switch  Criteria=u2 > Threshold
  "holder " : WBToolboxLibrary/Utilities/holder 
  holder 1 : WBToolboxLibrary/Utilities/holder 
  joints.smoothingTime : Constant  Value=Sm.smoothingTime_CoM_Joints(1)
  xCom : Subsystem
  CoM_des : Outport
  s_des : Outport  Port=2
  feet_in_contact : Outport  Port=3
  Kp_joints : Outport  Port=4
  state : Outport  Port=5
  nu_b + sDot : Outport  Port=6
  s : Outport  Port=7
  smoothingTime_CoM_Joints : Outport  Port=8
  Kp_CoM : Outport  Port=9
  Kd_CoM : Outport  Port=10
  w_H_b : Outport  Port=11
  wires:
  Constant/1 -> Switch1/2
  "holder "/1 -> s_des/1
  Switch1/1 -> CoM_des/1
  Mux/1 -> Switch1/3
  Constant2/1 -> Mux/2
  Constant3/1 -> Kp_joints/1
  Constant4/1 -> state/1
  Compute State Velocity/1(nu) -> nu_b + sDot/1
  holder 1/1 -> Mux/1, Reference Generator CoM/1(pos_CoM_0)
  Base to Fixed Link/1(fixed_link_H_b) -> Compute State Velocity/2(w_H_b), xCom/1(w_H_b), Reshape1/1
  xCom/1(x_CoM) -> holder 1/1
  joints.smoothingTime/1 -> smoothingTime_CoM_Joints/1
  joint_angles/1 -> Compute State Velocity/1(s), Base to Fixed Link/1(s), s/1, "holder "/1, xCom/2(s)
  Constant5/1 -> Kp_CoM/1
  Constant6/1 -> Kd_CoM/1
  Reshape1/1 -> w_H_b/1
  Constant1/1 -> Compute State Velocity/3(feet_in_contact), feet_in_contact/1
  IMU Measurements/1 -> Base to Fixed Link/2(inertial)
  Clock1/1 -> Reference Generator CoM/2(t)
  Reference Generator CoM/1(references_CoM) -> Switch1/1

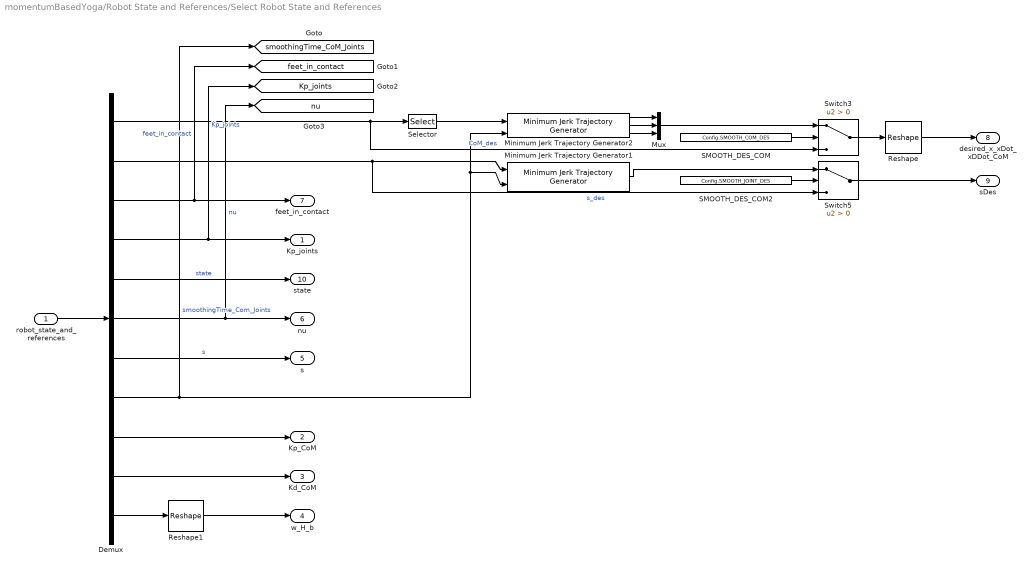
== system momentumBasedYoga/Robot State and References/Select Robot State and References ==
  robot_state_and_references : Inport
  Demux : Demux  Outputs=[9,ROBOT_DOF,2,ROBOT_DOF,1,ROBOT_DOF+6,ROBOT_DOF,1,3,3,16]
  Minimum Jerk Trajectory Generator1 : WBToolboxLibrary/Utilities/Minimum Jerk Trajectory Generator  externalSettlingTime=on  settlingTime=1  sampleTime=Config.T_STEP  resetOnSettlingTime=off  firstDerivatives=off  secondDerivatives=off  explicitInitialValue=off
  Minimum Jerk Trajectory Generator2 : WBToolboxLibrary/Utilities/Minimum Jerk Trajectory Generator  externalSettlingTime=on  settlingTime=references.com.smoothingTime  sampleTime=Config.T_STEP  resetOnSettlingTime=off  firstDerivatives=on  secondDerivatives=on  explicitInitialValue=off
  Mux : Mux  Inputs=3
  Reshape : Reshape  OutputDimensionality=Customize  OutputDimensions=[3,3]
  Reshape1 : Reshape  OutputDimensionality=Customize  OutputDimensions=[4;4]
  SMOOTH_DES_COM : Constant  Value=Config.SMOOTH_COM_DES
  SMOOTH_DES_COM2 : Constant  Value=Config.SMOOTH_JOINT_DES
  Selector : Selector  InputPortWidth=9  IndexOptions=Index vector (dialog)  Indices=[1 2 3]  OutputSizes=1
  Switch3 : Switch  Criteria=u2 > Threshold
  Switch5 : Switch  Criteria=u2 > Threshold
  Kp_joints : Outport
  Kp_CoM : Outport  Port=2
  Kd_CoM : Outport  Port=3
  w_H_b : Outport  Port=4
  s : Outport  Port=5
  nu : Outport  Port=6
  feet_in_contact : Outport  Port=7
  desired_x_xDot_xDDot_CoM : Outport  Port=8
  sDes : Outport  Port=9
  state : Outport  Port=10
  tag scope: Kp_joints=global, feet_in_contact=global, nu=global, smoothingTime_CoM_Joints=global
  wires:
  Reshape/1 -> desired_x_xDot_xDDot_CoM/1
  Minimum Jerk Trajectory Generator2/1 -> Mux/1
  Minimum Jerk Trajectory Generator2/2 -> Mux/2
  Switch3/1 -> Reshape/1
  Minimum Jerk Trajectory Generator2/3 -> Mux/3
  SMOOTH_DES_COM/1 -> Switch3/2
  SMOOTH_DES_COM2/1 -> Switch5/2
  Switch5/1 -> sDes/1
  Demux/7 -> s/1  "s"
  Demux/11 -> Reshape1/1
  Demux/5 -> state/1  "state"
  Demux/8 -> Minimum Jerk Trajectory Generator2/2, Minimum Jerk Trajectory Generator1/2, [smoothingTime_CoM_Joints]  "smoothingTime_Com_Joints"
  Mux/1 -> Switch3/1
  Selector/1 -> Minimum Jerk Trajectory Generator2/1
  Demux/2 -> Switch5/3, Minimum Jerk Trajectory Generator1/1  "s_des"
  Minimum Jerk Trajectory Generator1/1 -> Switch5/1
  Demux/6 -> [nu], nu/1  "nu"
  robot_state_and_references/1 -> Demux/1
  Demux/4 -> [Kp_joints], Kp_joints/1  "Kp_joints"
  Demux/3 -> [feet_in_contact], feet_in_contact/1  "feet_in_contact"
  Demux/9 -> Kp_CoM/1
  Demux/10 -> Kd_CoM/1
  Demux/1 -> Selector/1, Switch3/3  "CoM_des"
  Reshape1/1 -> w_H_b/1

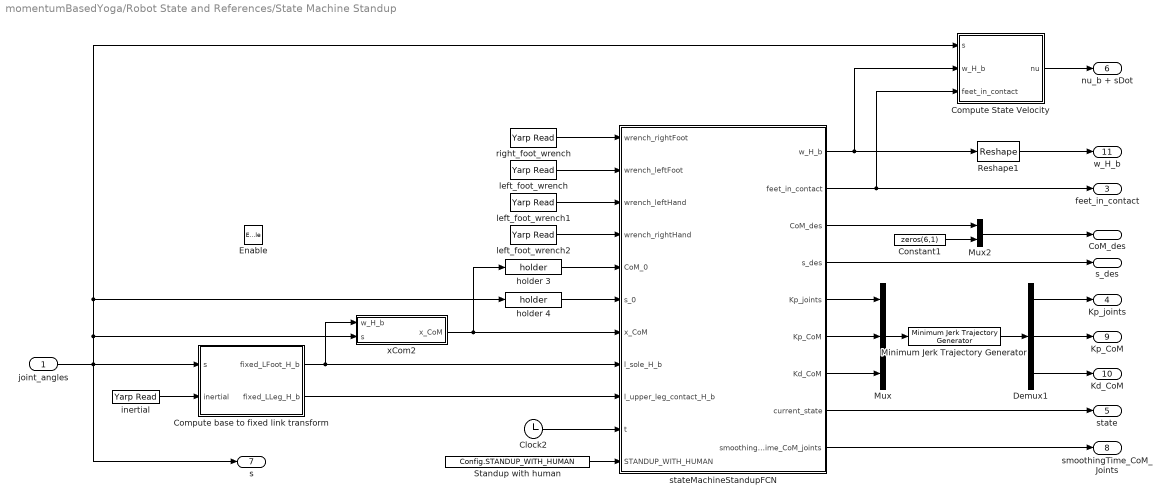
== system momentumBasedYoga/Robot State and References/State Machine Standup ==
  joint_angles : Inport
  Enable : EnablePort
  Clock2 : Clock
  Compute State Velocity : Subsystem
  Compute base to fixed link transform : Subsystem
  Constant1 : Constant  Value=zeros(6,1)
  Demux1 : Demux  Outputs=[ROBOT_DOF,3,3]
  Minimum Jerk Trajectory Generator : WBToolboxLibrary/Utilities/Minimum Jerk Trajectory Generator  externalSettlingTime=off  settlingTime=Gain.SmoothingTimeGainScheduling  sampleTime=Config.T_STEP  resetOnSettlingTime=off  firstDerivatives=off  secondDerivatives=off  explicitInitialValue=off
  Mux : Mux  Inputs=3
  Mux2 : Mux  Inputs=2
  Reshape1 : Reshape  OutputDimensions=[4;4]
  Standup with human : Constant  Value=Config.STANDUP_WITH_HUMAN
  holder 3 : WBToolboxLibrary/Utilities/holder 
  holder 4 : WBToolboxLibrary/Utilities/holder 
  inertial : WBToolboxLibrary/Utilities/Yarp Read  portName=Ports.IMU  signalSize=12  timeout=0.5  blocking=off  timestamp=off  autoconnect=on  errorOnConnection=off
  left_foot_wrench : WBToolboxLibrary/Utilities/Yarp Read  portName=Ports.WRENCH_LEFT_FOOT  signalSize=6  timeout=0.5  blocking=off  timestamp=off  autoconnect=on  errorOnConnection=on
  left_foot_wrench1 : WBToolboxLibrary/Utilities/Yarp Read  portName=Ports.LEFT_ARM  signalSize=6  timeout=0.5  blocking=off  timestamp=off  autoconnect=on  errorOnConnection=on
  left_foot_wrench2 : WBToolboxLibrary/Utilities/Yarp Read  portName=Ports.RIGHT_ARM  signalSize=6  timeout=0.5  blocking=off  timestamp=off  autoconnect=on  errorOnConnection=on
  right_foot_wrench : WBToolboxLibrary/Utilities/Yarp Read  portName=Ports.WRENCH_RIGHT_FOOT  signalSize=6  timeout=0.5  blocking=off  timestamp=off  autoconnect=on  errorOnConnection=on
  stateMachineStandupFCN : MATLAB Function  TreatAsAtomicUnit=on
  xCom2 : Subsystem
  CoM_des : Outport
  s_des : Outport  Port=2
  feet_in_contact : Outport  Port=3
  Kp_joints : Outport  Port=4
  state : Outport  Port=5
  nu_b + sDot : Outport  Port=6
  s : Outport  Port=7
  smoothingTime_CoM_Joints : Outport  Port=8
  Kp_CoM : Outport  Port=9
  Kd_CoM : Outport  Port=10
  w_H_b : Outport  Port=11
  wires:
  stateMachineStandupFCN/4(s_des) -> s_des/1
  stateMachineStandupFCN/3(CoM_des) -> Mux2/1
  Mux2/1 -> CoM_des/1
  Constant1/1 -> Mux2/2
  stateMachineStandupFCN/8(current_state) -> state/1
  stateMachineStandupFCN/2(feet_in_contact) -> feet_in_contact/1, Compute State Velocity/3(feet_in_contact)
  stateMachineStandupFCN/1(w_H_b) -> Reshape1/1, Compute State Velocity/2(w_H_b)
  Compute State Velocity/1(nu) -> nu_b + sDot/1
  stateMachineStandupFCN/9(smoothingTime_CoM_joints) -> smoothingTime_CoM_Joints/1
  stateMachineStandupFCN/6(Kp_CoM) -> Mux/2
  Demux1/3 -> Kd_CoM/1
  stateMachineStandupFCN/7(Kd_CoM) -> Mux/3
  stateMachineStandupFCN/5(Kp_joints) -> Mux/1
  Mux/1 -> Minimum Jerk Trajectory Generator/1
  Minimum Jerk Trajectory Generator/1 -> Demux1/1
  Demux1/1 -> Kp_joints/1
  Demux1/2 -> Kp_CoM/1
  inertial/1 -> Compute base to fixed link transform/2(inertial)
  Reshape1/1 -> w_H_b/1
  right_foot_wrench/1 -> stateMachineStandupFCN/1(wrench_rightFoot)
  left_foot_wrench/1 -> stateMachineStandupFCN/2(wrench_leftFoot)
  left_foot_wrench2/1 -> stateMachineStandupFCN/4(wrench_rightHand)
  left_foot_wrench1/1 -> stateMachineStandupFCN/3(wrench_leftHand)
  xCom2/1(x_CoM) -> stateMachineStandupFCN/7(x_CoM), holder 3/1
  Compute base to fixed link transform/2(fixed_LLeg_H_b) -> stateMachineStandupFCN/9(l_upper_leg_contact_H_b)
  holder 3/1 -> stateMachineStandupFCN/5(CoM_0)
  Clock2/1 -> stateMachineStandupFCN/10(t)
  Standup with human/1 -> stateMachineStandupFCN/11(STANDUP_WITH_HUMAN)
  holder 4/1 -> stateMachineStandupFCN/6(s_0)
  joint_angles/1 -> Compute State Velocity/1(s), holder 4/1, xCom2/2(s), Compute base to fixed link transform/1(s), s/1
  Compute base to fixed link transform/1(fixed_LFoot_H_b) -> stateMachineStandupFCN/8(l_sole_H_b), xCom2/1(w_H_b)

== system momentumBasedYoga/synchronizer/GAZEBO_SYNCHRONIZER ==
  Enable : EnablePort
  Simulator Synchronizer : WBToolboxLibrary/Utilities/Simulator Synchronizer  period=Config.T_STEP  serverPortName='/clock/rpc'  clientPortName='/WBT_synchronizer/rpc:o'

== system momentumBasedYoga/synchronizer/REAL_TIME_SYNC ==
  Enable : EnablePort
  Real Time Synchronizer : WBToolboxLibrary/Utilities/Real Time Synchronizer  period=Config.T_STEP

== system momentumBasedYoga/Balancing Controller QP/Approximate Momentum Integral/Compute base to fixed link transform ==
  s : Inport
  inertial : Inport  Port=2
  Constant7 : Constant  Value=eye(4)
  "Floating Base to Fixed Link Transform (Left Foot) " : Subsystem
  Floating Base to Fixed Link Transform (Right Foot) : Subsystem
  LFoot to World Transform with Fixed Base : WBToolboxLibrary/wholeBodyModel/Kinematics/Forward Kinematics  frameName=Frames.LEFT_FOOT
  RFoot to World Transform with Fixed Base : WBToolboxLibrary/wholeBodyModel/Kinematics/Forward Kinematics  frameName=Frames.RIGHT_FOOT
  fixed_LFoot_H_b : Outport
  fixed_RFoot_H_b : Outport  Port=2
  wires:
  Constant7/1 -> RFoot to World Transform with Fixed Base/1, LFoot to World Transform with Fixed Base/1
  s/1 -> "Floating Base to Fixed Link Transform (Left Foot) "/1(s), Floating Base to Fixed Link Transform (Right Foot)/1(s), LFoot to World Transform with Fixed Base/2, RFoot to World Transform with Fixed Base/2
  "Floating Base to Fixed Link Transform (Left Foot) "/1(fixed_link_H_b) -> fixed_LFoot_H_b/1
  Floating Base to Fixed Link Transform (Right Foot)/1(fixed_link_H_b) -> fixed_RFoot_H_b/1
  RFoot to World Transform with Fixed Base/1 -> Floating Base to Fixed Link Transform (Right Foot)/3(w_H_fixed_link)
  LFoot to World Transform with Fixed Base/1 -> "Floating Base to Fixed Link Transform (Left Foot) "/3(w_H_fixed_link)
  inertial/1 -> "Floating Base to Fixed Link Transform (Left Foot) "/2(inertial), Floating Base to Fixed Link Transform (Right Foot)/2(inertial)

== system momentumBasedYoga/Balancing Controller QP/Compute Motor Torques/QP Solver ==
  feet_in_contact : Inport
  HessianMatrix_QP1Foot : Inport  Port=2
  gradient_QP1Foot : Inport  Port=3
  ConstraintsMatrix_QP1Foot : Inport  Port=4
  bVectorConstraints_QP1Foot : Inport  Port=5
  HessianMatrix_QP2Feet : Inport  Port=6
  gradient_QP2Feet : Inport  Port=7
  ConstraintsMatrix_QP2Feet : Inport  Port=8
  bVectorConstraints_Qp2Feet : Inport  Port=9
  Constant1 : Constant  Value=Config.USE_QP_SOLVER
  Level-2 MATLAB S-Function : M-S-Function  FunctionName=QPBalancingYoga
  f_one_foot : Outport
  f0_two_feet : Outport  Port=2
  tag scope: exit_flag_QP=global
  wires:
  Level-2 MATLAB S-Function/1 -> f0_two_feet/1
  HessianMatrix_QP1Foot/1 -> Level-2 MATLAB S-Function/7
  gradient_QP1Foot/1 -> Level-2 MATLAB S-Function/8
  ConstraintsMatrix_QP1Foot/1 -> Level-2 MATLAB S-Function/9
  bVectorConstraints_QP1Foot/1 -> Level-2 MATLAB S-Function/10
  Level-2 MATLAB S-Function/3 -> f_one_foot/1
  feet_in_contact/1 -> Level-2 MATLAB S-Function/1
  HessianMatrix_QP2Feet/1 -> Level-2 MATLAB S-Function/2
  gradient_QP2Feet/1 -> Level-2 MATLAB S-Function/3
  ConstraintsMatrix_QP2Feet/1 -> Level-2 MATLAB S-Function/4
  bVectorConstraints_Qp2Feet/1 -> Level-2 MATLAB S-Function/5
  Constant1/1 -> Level-2 MATLAB S-Function/6
  Level-2 MATLAB S-Function/2 -> [exit_flag_QP]  "exit flag QP"

== system momentumBasedYoga/Dynamics and Kinematics/Dynamics Variables/Add Motors Reflected Inertia ==
  M : Inport
  Add Motor Reflected Inertia : MATLAB Function  TreatAsAtomicUnit=on
  M_with_motor_inertia : Outport
  wires:
  M/1 -> Add Motor Reflected Inertia/1(M)
  Add Motor Reflected Inertia/1(M_with_inertia) -> M_with_motor_inertia/1

== system momentumBasedYoga/Dynamics and Kinematics/Kinematics Variables/Arm External Forces ==
  w_H_b : Inport
  s : Inport  Port=2
  r_sole1 : WBToolboxLibrary/wholeBodyModel/Kinematics/Forward Kinematics  frameName=Frames.RIGHT_HAND
  r_sole2 : WBToolboxLibrary/wholeBodyModel/Kinematics/Forward Kinematics  frameName=Frames.LEFT_HAND
  w_H_LArm : Outport
  w_H_RArm : Outport  Port=2
  wires:
  s/1 -> r_sole2/2, r_sole1/2
  r_sole1/1 -> w_H_RArm/1
  w_H_b/1 -> r_sole2/1, r_sole1/1
  r_sole2/1 -> w_H_LArm/1

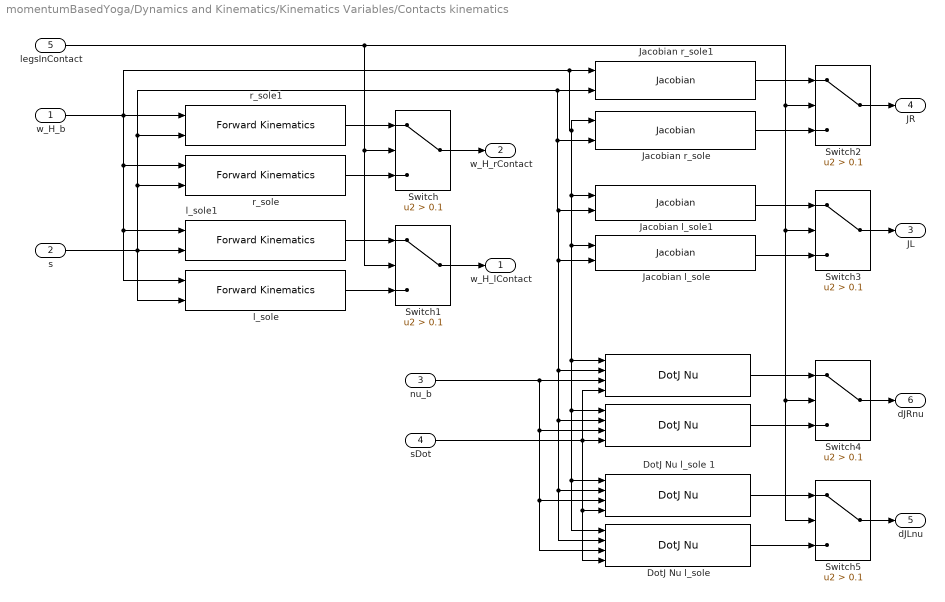
== system momentumBasedYoga/Dynamics and Kinematics/Kinematics Variables/Contacts kinematics ==
  w_H_b : Inport
  s : Inport  Port=2
  nu_b : Inport  Port=3
  sDot : Inport  Port=4
  legsInContact : Inport  Port=5
  " " : WBToolboxLibrary/wholeBodyModel/Jacobians/DotJ Nu  frameName=Frames.RIGHT_LEG
  "    " : WBToolboxLibrary/wholeBodyModel/Jacobians/DotJ Nu  frameName=Frames.RIGHT_FOOT
  "DotJ Nu l_sole " : WBToolboxLibrary/wholeBodyModel/Jacobians/DotJ Nu  frameName=Frames.LEFT_FOOT
  DotJ Nu l_sole 1 : WBToolboxLibrary/wholeBodyModel/Jacobians/DotJ Nu  frameName=Frames.LEFT_LEG
  Jacobian l_sole : WBToolboxLibrary/wholeBodyModel/Jacobians/Jacobian  frameName=Frames.LEFT_FOOT
  Jacobian l_sole1 : WBToolboxLibrary/wholeBodyModel/Jacobians/Jacobian  frameName=Frames.LEFT_LEG
  Jacobian r_sole : WBToolboxLibrary/wholeBodyModel/Jacobians/Jacobian  frameName=Frames.RIGHT_FOOT
  Jacobian r_sole1 : WBToolboxLibrary/wholeBodyModel/Jacobians/Jacobian  frameName=Frames.RIGHT_LEG
  Switch{,1..5} (6 alike) : Switch  Criteria=u2 > Threshold  Threshold=0.1
  l_sole : WBToolboxLibrary/wholeBodyModel/Kinematics/Forward Kinematics  frameName=Frames.LEFT_FOOT
  l_sole1 : WBToolboxLibrary/wholeBodyModel/Kinematics/Forward Kinematics  frameName=Frames.LEFT_LEG
  r_sole : WBToolboxLibrary/wholeBodyModel/Kinematics/Forward Kinematics  frameName=Frames.RIGHT_FOOT
  r_sole1 : WBToolboxLibrary/wholeBodyModel/Kinematics/Forward Kinematics  frameName=Frames.RIGHT_LEG
  w_H_lContact : Outport
  w_H_rContact : Outport  Port=2
  JL : Outport  Port=3
  JR : Outport  Port=4
  dJLnu : Outport  Port=5
  dJRnu : Outport  Port=6
  wires:
  r_sole1/1 -> Switch/1
  r_sole/1 -> Switch/3
  l_sole1/1 -> Switch1/1
  l_sole/1 -> Switch1/3
  Switch1/1 -> w_H_lContact/1
  Switch/1 -> w_H_rContact/1
  w_H_b/1 -> Jacobian l_sole1/1, "DotJ Nu l_sole "/1, DotJ Nu l_sole 1/1, "    "/1, " "/1, Jacobian l_sole/1, Jacobian r_sole/1, Jacobian r_sole1/1, r_sole1/1, l_sole/1, l_sole1/1, r_sole/1
  Jacobian r_sole1/1 -> Switch2/1
  legsInContact/1 -> Switch1/2, Switch/2, Switch5/2, Switch4/2, Switch3/2, Switch2/2
  Jacobian r_sole/1 -> Switch2/3
  Jacobian l_sole1/1 -> Switch3/1
  Jacobian l_sole/1 -> Switch3/3
  Switch2/1 -> JR/1
  Switch3/1 -> JL/1
  s/1 -> l_sole/2, "DotJ Nu l_sole "/2, DotJ Nu l_sole 1/2, "    "/2, " "/2, Jacobian l_sole/2, Jacobian l_sole1/2, Jacobian r_sole/2, Jacobian r_sole1/2, r_sole1/2, r_sole/2, l_sole1/2
  nu_b/1 -> "DotJ Nu l_sole "/3, DotJ Nu l_sole 1/3, "    "/3, " "/3
  sDot/1 -> "DotJ Nu l_sole "/4, DotJ Nu l_sole 1/4, " "/4, "    "/4
  " "/1 -> Switch4/1
  "    "/1 -> Switch4/3
  DotJ Nu l_sole 1/1 -> Switch5/1
  Switch4/1 -> dJRnu/1
  Switch5/1 -> dJLnu/1
  "DotJ Nu l_sole "/1 -> Switch5/3

== system momentumBasedYoga/Dynamics and Kinematics/Kinematics Variables/xCom ==
  w_H_b : Inport
  s : Inport  Port=2
  CoM : WBToolboxLibrary/wholeBodyModel/Kinematics/Forward Kinematics  frameName=Frames.COM
  "CoM6D ->  CoMXYZ2" : Selector  NumberOfDimensions=2  InputPortWidth=7  IndexOptions=Index vector (dialog),Index vector (dialog)  Indices=[1 2 3],[4]  OutputSizes=1,1
  x_CoM : Outport
  wires:
  s/1 -> CoM/2
  "CoM6D ->  CoMXYZ2"/1 -> x_CoM/1
  CoM/1 -> "CoM6D ->  CoMXYZ2"/1
  w_H_b/1 -> CoM/1

== system momentumBasedYoga/Robot State and References/Internal Coordinator/Base to Fixed Link ==
  s : Inport
  inertial : Inport  Port=2
  Fixed Link to World Transform : Subsystem
  "Floating Base to Fixed Link Transform " : Subsystem
  fixed_link_H_b : Outport
  wires:
  "Floating Base to Fixed Link Transform "/1(fixed_link_H_b) -> fixed_link_H_b/1
  inertial/1 -> "Floating Base to Fixed Link Transform "/2(inertial)
  s/1 -> Fixed Link to World Transform/1(s), "Floating Base to Fixed Link Transform "/1(s)
  Fixed Link to World Transform/1(w_H_fixed_link) -> "Floating Base to Fixed Link Transform "/3(w_H_fixed_link)

== system momentumBasedYoga/Robot State and References/Internal Coordinator/Compute State Velocity ==
  s : Inport
  w_H_b : Inport  Port=2
  feet_in_contact : Inport  Port=3
  Compute Base Velocity : MATLAB Function  TreatAsAtomicUnit=on
  Feet Jacobians : Subsystem
  Get Measurement : WBToolboxLibrary/wholeBodyStates/Get Measurement  measuredType=Joints Velocity
  Mux : Mux  Inputs=2
  nu : Outport
  wires:
  Get Measurement/1 -> Mux/2, Compute Base Velocity/4(sDot)
  Mux/1 -> nu/1
  feet_in_contact/1 -> Compute Base Velocity/3(feet_in_contact)
  Compute Base Velocity/1(nu_b) -> Mux/1
  s/1 -> Feet Jacobians/1(s)
  w_H_b/1 -> Feet Jacobians/2(w_H_b)
  Feet Jacobians/1(J_LFoot) -> Compute Base Velocity/1(J_LeftFoot)
  Feet Jacobians/2(J_RFoot) -> Compute Base Velocity/2(J_RightFoot)

== system momentumBasedYoga/Robot State and References/Internal Coordinator/xCom ==
  w_H_b : Inport
  s : Inport  Port=2
  CoM : WBToolboxLibrary/wholeBodyModel/Kinematics/Forward Kinematics  frameName=Frames.COM
  "CoM6D ->  CoMXYZ2" : Selector  NumberOfDimensions=2  InputPortWidth=7  IndexOptions=Index vector (dialog),Index vector (dialog)  Indices=[1 2 3],[4]  OutputSizes=1,1
  x_CoM : Outport
  wires:
  s/1 -> CoM/2
  "CoM6D ->  CoMXYZ2"/1 -> x_CoM/1
  CoM/1 -> "CoM6D ->  CoMXYZ2"/1
  w_H_b/1 -> CoM/1

== system momentumBasedYoga/Robot State and References/State Machine Standup/Compute State Velocity ==
  s : Inport
  w_H_b : Inport  Port=2
  feet_in_contact : Inport  Port=3
  Compute Base Velocity : MATLAB Function  TreatAsAtomicUnit=on
  Feet Jacobians : Subsystem
  Get Measurement : WBToolboxLibrary/wholeBodyStates/Get Measurement  measuredType=Joints Velocity
  Mux : Mux  Inputs=2
  nu : Outport
  wires:
  Get Measurement/1 -> Mux/2, Compute Base Velocity/4(sDot)
  Mux/1 -> nu/1
  feet_in_contact/1 -> Compute Base Velocity/3(feet_in_contact)
  Compute Base Velocity/1(nu_b) -> Mux/1
  s/1 -> Feet Jacobians/1(s)
  w_H_b/1 -> Feet Jacobians/2(w_H_b)
  Feet Jacobians/1(J_LFoot) -> Compute Base Velocity/1(J_LeftFoot)
  Feet Jacobians/2(J_RFoot) -> Compute Base Velocity/2(J_RightFoot)
